simulink model "LevelshiftPWM"  (R2023b)
settings: Solver=ode4  StartTime=0.0  StopTime=0.1  FixedStep=1e-5  RelTol=1e-3
libraries: simulink x12, spspowerguiLib x1
settings Model: Creator=user  LastModifiedBy=user

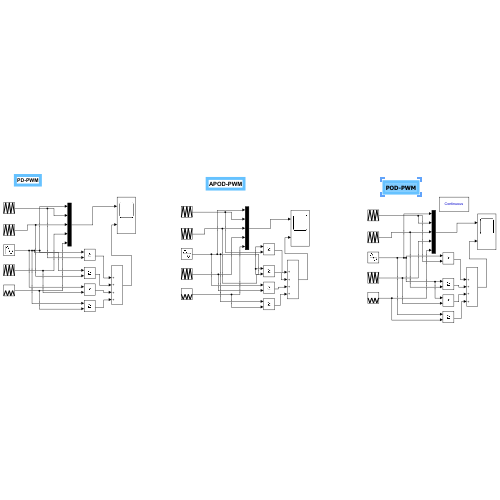
[thumbnail: Simulink's stored preview of the top-level diagram]
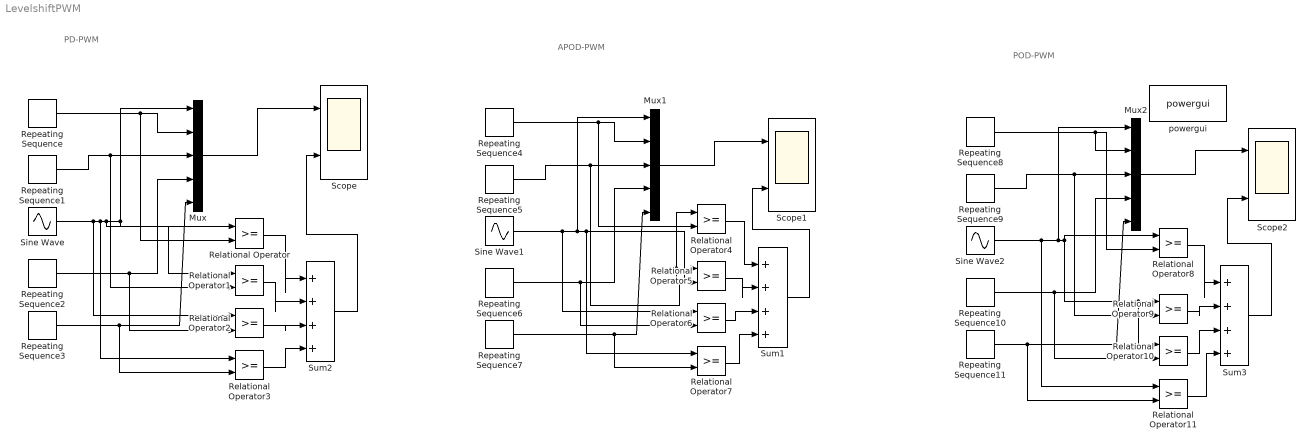
== system LevelshiftPWM ==
  note: POD-PWM
  note: APOD-PWM
  note: PD-PWM
  Mux : Mux  Inputs=5
  Mux1 : Mux  Inputs=5
  Mux2 : Mux  Inputs=5
  Relational Operator{,1..11} (12 alike) : RelationalOperator  OutDataTypeStr=boolean  RndMeth=Simplest  InputSameDT=off
  Repeating Sequence : simulink/Sources/Repeating Sequence  rep_seq_t=[0 1 2]*[1/1000]  rep_seq_y=[1 2 1]
  Repeating Sequence1 : simulink/Sources/Repeating Sequence  rep_seq_t=[0 1 2]*[1/1000]  rep_seq_y=[0 1 0]
  Repeating Sequence10 : simulink/Sources/Repeating Sequence  rep_seq_t=[0 1 2]*[1/1000]  rep_seq_y=[0 -1 0]
  Repeating Sequence11 : simulink/Sources/Repeating Sequence  rep_seq_t=[0 1 2]*[1/1000]  rep_seq_y=[-1 -2 -1]
  Repeating Sequence2 : simulink/Sources/Repeating Sequence  rep_seq_t=[0 1 2]*[1/1000]  rep_seq_y=[-1 0 -1]
  Repeating Sequence3 : simulink/Sources/Repeating Sequence  rep_seq_t=[0 1 2]*[1/1000]  rep_seq_y=[-2 -1 -2]
  Repeating Sequence4 : simulink/Sources/Repeating Sequence  rep_seq_t=[0 1 2]*[1/1000]  rep_seq_y=[1 2 1]
  Repeating Sequence5 : simulink/Sources/Repeating Sequence  rep_seq_t=[0 1 2]*[1/1000]  rep_seq_y=[1 0 1]
  Repeating Sequence6 : simulink/Sources/Repeating Sequence  rep_seq_t=[0 1 2]*[1/1000]  rep_seq_y=[-1 0 -1]
  Repeating Sequence7 : simulink/Sources/Repeating Sequence  rep_seq_t=[0 1 2]*[1/1000]  rep_seq_y=[-1 -2 -1]
  Repeating Sequence8 : simulink/Sources/Repeating Sequence  rep_seq_t=[0 1 2]*[1/1000]  rep_seq_y=[1 2 1]
  Repeating Sequence9 : simulink/Sources/Repeating Sequence  rep_seq_t=[0 1 2]*[1/1000]  rep_seq_y=[0 1 0]
  Scope : Scope  NumInputPorts=2
  Scope1 : Scope  NumInputPorts=2
  Scope2 : Scope  NumInputPorts=2
  Sine Wave : Sin  Amplitude=2  Frequency=2*pi*50  SampleTime=0
  Sine Wave1 : Sin  Amplitude=2  Frequency=2*pi*50  SampleTime=0
  Sine Wave2 : Sin  Amplitude=2  Frequency=2*pi*50  SampleTime=0
  Sum1 : Sum  Inputs=|++++
  Sum2 : Sum  Inputs=|++++
  Sum3 : Sum  Inputs=|++++
  powergui : spspowerguiLib/powergui  Priority=1  SimulationMode=Continuous  SampleTime=1e-5  frequency=60  Iterations=50  frequencyindice=60  Pbase=100e6  ErrMax=1e-4  UnitsV=kV  UnitsW=MW  buscounter=0  FunctionMessages=off  echomessages=off  EnableUseOfTLC=off  CurrentSourceSwitches=off  DisableSnubberDevices=off  DisableRonSwitches=off  DisableVfSwitches=off  DisplayEquations=off  AutomaticDiscreteSolvers=off  SolverType=Tustin/Backward Euler (TBE)  Interpol=off  ExternalGateDelay=off  methode=off  Ts=100  x0status=blocks  SPID=on  SwTol=0  HookPort=off  NonlinearTolerance=1e-4  nMaxIteration=100  ContinueOnMaxIteration=off  RestoreLinks=warning  ResistiveCurrentMeasurement=off  Frange=[0:2:500]  Ylog=off  Xlog=on  ShowGrid=off  save=off  variable=ZData  structure=0  ZoomFFT=off  StartTime=0.0  cycles=1  DisplayStyle=1  fundamental=60  FreqAxis=off  MaxFrequency=1000  frequencyindicesteady=1  RmsSteady=1  display=off
  wires:
  Sine Wave/1 -> Relational Operator2/1, Relational Operator3/1, Relational Operator1/1, Mux/1, Relational Operator/1
  Repeating Sequence/1 -> Relational Operator/2, Mux/2
  Repeating Sequence1/1 -> Relational Operator1/2, Mux/3
  Repeating Sequence3/1 -> Relational Operator3/2, Mux/5
  Repeating Sequence2/1 -> Relational Operator2/2, Mux/4
  Mux/1 -> Scope/1
  Mux1/1 -> Scope1/1
  Mux2/1 -> Scope2/1
  Relational Operator/1 -> Sum2/1
  Relational Operator1/1 -> Sum2/2
  Relational Operator2/1 -> Sum2/3
  Relational Operator3/1 -> Sum2/4
  Sum2/1 -> Scope/2
  Relational Operator6/1 -> Sum1/3
  Relational Operator4/1 -> Sum1/1
  Repeating Sequence7/1 -> Relational Operator7/2, Mux1/5
  Repeating Sequence4/1 -> Relational Operator4/2, Mux1/2
  Relational Operator7/1 -> Sum1/4
  Repeating Sequence5/1 -> Relational Operator5/2, Mux1/3
  Relational Operator5/1 -> Sum1/2
  Sine Wave1/1 -> Relational Operator6/1, Relational Operator7/1, Relational Operator5/1, Relational Operator4/1, Mux1/1
  Sum1/1 -> Scope1/2
  Repeating Sequence6/1 -> Relational Operator6/2, Mux1/4
  Relational Operator10/1 -> Sum3/3
  Relational Operator8/1 -> Sum3/1
  Repeating Sequence11/1 -> Relational Operator11/2, Mux2/5
  Repeating Sequence8/1 -> Relational Operator8/2, Mux2/2
  Relational Operator11/1 -> Sum3/4
  Repeating Sequence9/1 -> Relational Operator9/2, Mux2/3
  Relational Operator9/1 -> Sum3/2
  Sine Wave2/1 -> Relational Operator11/1, Relational Operator10/1, Relational Operator9/1, Relational Operator8/1, Mux2/1
  Sum3/1 -> Scope2/2
  Repeating Sequence10/1 -> Relational Operator10/2, Mux2/4
